simulink model "Super11"  (Simulink 8.7)
settings: Solver=FixedStepDiscrete  StartTime=0.0  StopTime=10.0  RelTol=1e-3
settings Model: Creator=scaife  LastModifiedBy=bourbouh  ExtModeAutoUpdateStatusClock=off
settings DataIOCC: SignalLoggingSaveFormat=ModelDataLogs  SignalLoggingName=sigsOut
settings DebuggingCC: SaveWithParameterizedLinksMsg=none  SignalResolutionControl=TryResolveAllWithWarning  MultiTaskDSMMsg=warning  MultiTaskCondExecSysMsg=none
settings HardwareCC: TargetUnknown=on
settings SFSimCC: SimParseCustomCode=off
settings GRTTargetCC: CombineOutputUpdateFcns=off  GRTInterface=on

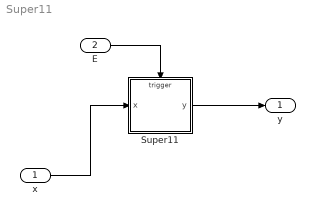
== system Super11 ==
  x : Inport
  E : Inport  Port=2
  Super11 : Stateflow chart  TreatAsAtomicUnit=on
  y : Outport
  wires:
  x/1 -> Super11/1(x)
  Super11/1(y) -> y/1
  E/1 -> Super11/Trigger

== stateflow chart Super11 ==
  state A
    du : y++;
  state B
    du : y++;
    state B1
      du : y++;
    state B2
      du : y++;
      state B2a
        du : y++;
      (default) -> B2a
      B2a -> (junction 11) : E
    (default) -> B1
    B1 -> B2 : E
    (junction 11) -> B1 [order 2] : [x<>0]
  (junction 17) -> B [order 1] : [x==0]
  A -> (junction 17) : E
  (junction 17) -> B2a [order 2] : [x<>0]
  (junction 11) -> A [order 1] : [x==0]
  (default) -> A
  data: x input int8; y output uint32
  events: E input EITHER_EDGE_EVENT
